simulink subsystem "rss_MotoTempSensFaltDia"  (R2023a)
settings: Solver=VariableStepAuto  StartTime=0.0  StopTime=10.0  RelTol=1e-3
undefined symbols (not defined in the file): ENM_TYPE_FALT, Gu16_ctMotoTempFaltConfCnt_C, Gu16_ctMotoTempFaltRcvyCnt_C, Gu16_uADMotoTempFaltHiLim_C, Gu16_uADMotoTempFaltLoLim_C
libraries: lib_debounce x1, lib_fault_definiteness x1
settings Model: Creator=xiaoqiang.yuan  LastModifiedBy=xiaoqiang.yuan

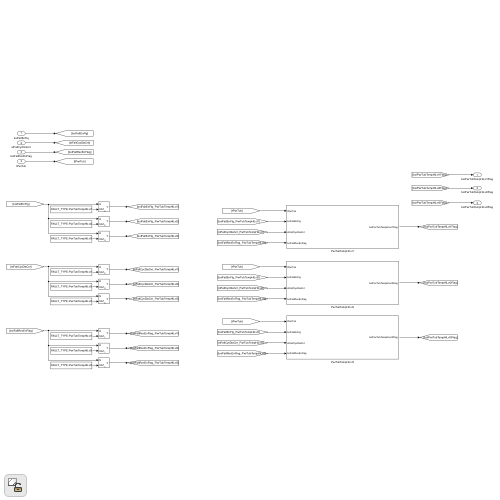
[thumbnail: Simulink's stored preview of the top-level diagram]
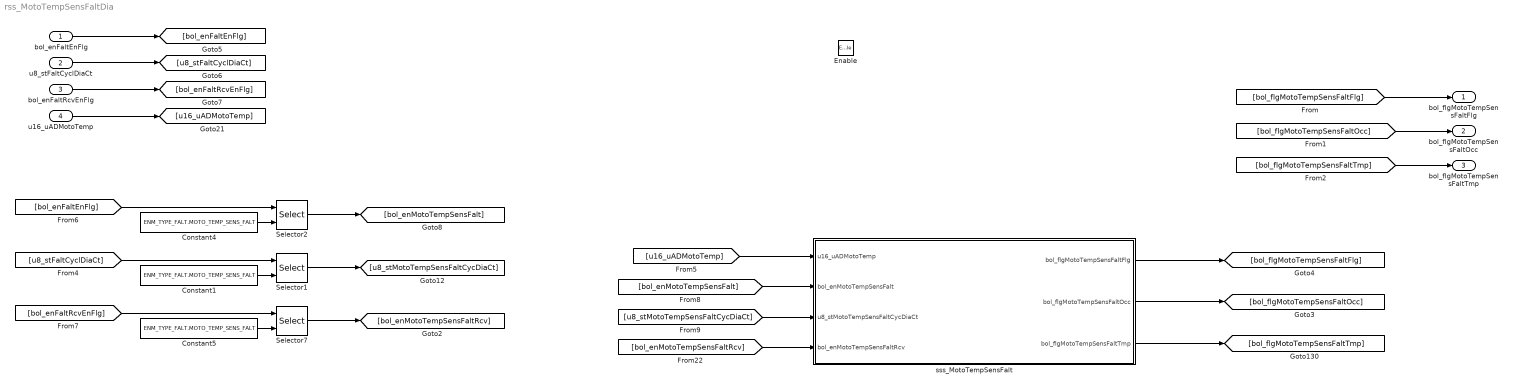
== system rss_MotoTempSensFaltDia ==
  bol_enFaltEnFlg : Inport  OutDataTypeStr=boolean
  u8_stFaltCyclDiaCt : Inport  Port=2  OutDataTypeStr=uint8
  bol_enFaltRcvEnFlg : Inport  Port=3  OutDataTypeStr=boolean
  u16_uADMotoTemp : Inport  Port=4  OutDataTypeStr=uint16
  Enable : EnablePort
  Constant1 : Constant  Value=ENM_TYPE_FALT.MOTO_TEMP_SENS_FALT
  Constant4 : Constant  Value=ENM_TYPE_FALT.MOTO_TEMP_SENS_FALT
  Constant5 : Constant  Value=ENM_TYPE_FALT.MOTO_TEMP_SENS_FALT
  Selector1 : Selector  IndexMode=Zero-based  InputPortWidth=Cdbl_numFaltDiaNum  IndexOptions=Index vector (port)  Indices=[1 3]  OutputSizes=1
  Selector2 : Selector  IndexMode=Zero-based  InputPortWidth=Cdbl_numFaltDiaNum  IndexOptions=Index vector (port)  Indices=[1 3]  OutputSizes=1
  Selector7 : Selector  IndexMode=Zero-based  InputPortWidth=Cdbl_numFaltDiaNum  IndexOptions=Index vector (port)  Indices=[1 3]  OutputSizes=1
  sss_MotoTempSensFalt : Subsystem
  bol_flgMotoTempSensFaltFlg : Outport  OutDataTypeStr=boolean
  bol_flgMotoTempSensFaltOcc : Outport  Port=2  OutDataTypeStr=boolean
  bol_flgMotoTempSensFaltTmp : Outport  Port=3  OutDataTypeStr=boolean
  wires:
  [bol_flgMotoTempSensFaltFlg] -> bol_flgMotoTempSensFaltFlg/1
  u16_uADMotoTemp/1 -> [u16_uADMotoTemp]
  Selector2/1 -> [bol_enMotoTempSensFalt]
  [bol_enFaltEnFlg] -> Selector2/1
  [bol_enMotoTempSensFalt] -> sss_MotoTempSensFalt/2(bol_enMotoTempSensFalt)
  Constant4/1 -> Selector2/2
  [u8_stMotoTempSensFaltCycDiaCt] -> sss_MotoTempSensFalt/3(u8_stMotoTempSensFaltCycDiaCt)
  [u16_uADMotoTemp] -> sss_MotoTempSensFalt/1(u16_uADMotoTemp)
  bol_enFaltEnFlg/1 -> [bol_enFaltEnFlg]
  bol_enFaltRcvEnFlg/1 -> [bol_enFaltRcvEnFlg]
  u8_stFaltCyclDiaCt/1 -> [u8_stFaltCyclDiaCt]
  [bol_enMotoTempSensFaltRcv] -> sss_MotoTempSensFalt/4(bol_enMotoTempSensFaltRcv)
  Selector1/1 -> [u8_stMotoTempSensFaltCycDiaCt]
  Constant1/1 -> Selector1/2
  [u8_stFaltCyclDiaCt] -> Selector1/1
  Selector7/1 -> [bol_enMotoTempSensFaltRcv]
  Constant5/1 -> Selector7/2
  [bol_enFaltRcvEnFlg] -> Selector7/1
  sss_MotoTempSensFalt/1(bol_flgMotoTempSensFaltFlg) -> [bol_flgMotoTempSensFaltFlg]
  sss_MotoTempSensFalt/2(bol_flgMotoTempSensFaltOcc) -> [bol_flgMotoTempSensFaltOcc]
  [bol_flgMotoTempSensFaltOcc] -> bol_flgMotoTempSensFaltOcc/1
  [bol_flgMotoTempSensFaltTmp] -> bol_flgMotoTempSensFaltTmp/1
  sss_MotoTempSensFalt/3(bol_flgMotoTempSensFaltTmp) -> [bol_flgMotoTempSensFaltTmp]

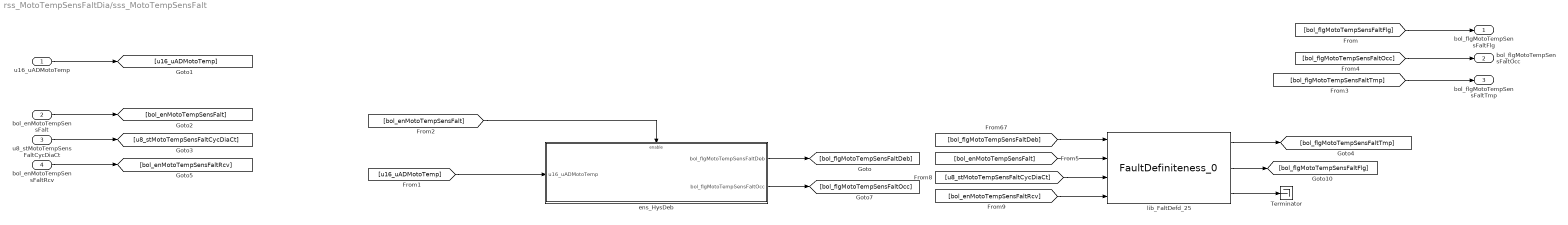
== system rss_MotoTempSensFaltDia/sss_MotoTempSensFalt ==
  u16_uADMotoTemp : Inport
  bol_enMotoTempSensFalt : Inport  Port=2
  u8_stMotoTempSensFaltCycDiaCt : Inport  Port=3
  bol_enMotoTempSensFaltRcv : Inport  Port=4
  Terminator : Terminator
  ens_HysDeb : Subsystem
  lib_FaltDefd_25 : lib_fault_definiteness/FaultDefiniteness_0  lb_FaltWaitRecvCnt=Gu16_ctMotoTempFaltConfCnt_C
  bol_flgMotoTempSensFaltFlg : Outport
  bol_flgMotoTempSensFaltOcc : Outport  Port=2
  bol_flgMotoTempSensFaltTmp : Outport  Port=3  OutDataTypeStr=boolean
  wires:
  [bol_flgMotoTempSensFaltTmp] -> bol_flgMotoTempSensFaltTmp/1
  [bol_flgMotoTempSensFaltOcc] -> bol_flgMotoTempSensFaltOcc/1
  ens_HysDeb/2(bol_flgMotoTempSensFaltOcc) -> [bol_flgMotoTempSensFaltOcc]
  lib_FaltDefd_25/1 -> [bol_flgMotoTempSensFaltTmp]
  lib_FaltDefd_25/2 -> [bol_flgMotoTempSensFaltFlg]
  lib_FaltDefd_25/3 -> Terminator/1
  [bol_enMotoTempSensFalt] -> ens_HysDeb/Enable
  [u16_uADMotoTemp] -> ens_HysDeb/1(u16_uADMotoTemp)
  ens_HysDeb/1(bol_flgMotoTempSensFaltDeb) -> [bol_flgMotoTempSensFaltDeb]
  bol_enMotoTempSensFaltRcv/1 -> [bol_enMotoTempSensFaltRcv]
  u8_stMotoTempSensFaltCycDiaCt/1 -> [u8_stMotoTempSensFaltCycDiaCt]
  bol_enMotoTempSensFalt/1 -> [bol_enMotoTempSensFalt]
  [bol_flgMotoTempSensFaltFlg] -> bol_flgMotoTempSensFaltFlg/1
  u16_uADMotoTemp/1 -> [u16_uADMotoTemp]
  [bol_enMotoTempSensFaltRcv] -> lib_FaltDefd_25/4
  [u8_stMotoTempSensFaltCycDiaCt] -> lib_FaltDefd_25/3
  [bol_enMotoTempSensFalt] -> lib_FaltDefd_25/2
  [bol_flgMotoTempSensFaltDeb] -> lib_FaltDefd_25/1

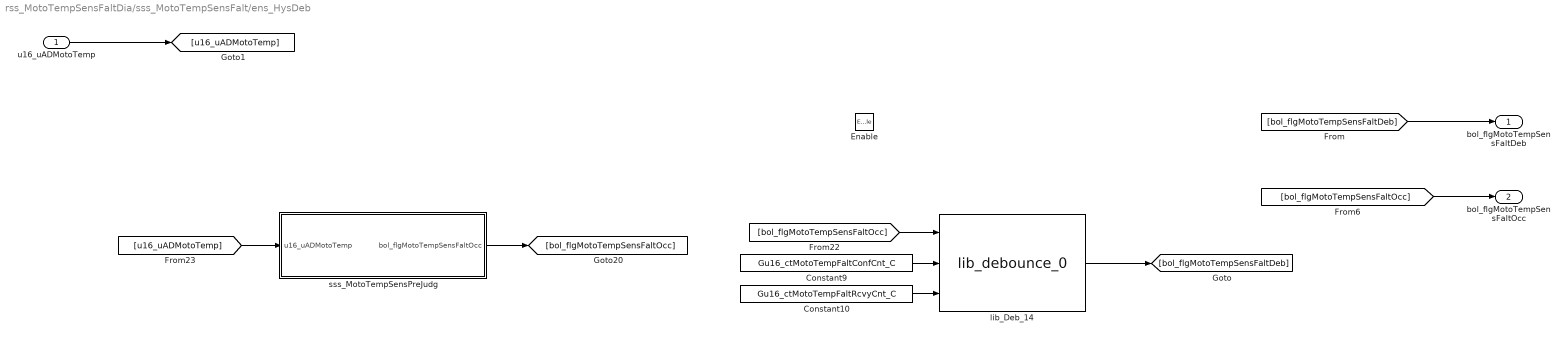
== system rss_MotoTempSensFaltDia/sss_MotoTempSensFalt/ens_HysDeb ==
  u16_uADMotoTemp : Inport
  Enable : EnablePort
  Constant10 : Constant  Value=Gu16_ctMotoTempFaltRcvyCnt_C
  Constant9 : Constant  Value=Gu16_ctMotoTempFaltConfCnt_C
  lib_Deb_14 : lib_debounce/lib_debounce_0
  sss_MotoTempSensPreJudg : Subsystem
  bol_flgMotoTempSensFaltDeb : Outport
  bol_flgMotoTempSensFaltOcc : Outport  Port=2
  wires:
  lib_Deb_14/1 -> [bol_flgMotoTempSensFaltDeb]
  [bol_flgMotoTempSensFaltOcc] -> lib_Deb_14/1
  Constant9/1 -> lib_Deb_14/2
  sss_MotoTempSensPreJudg/1(bol_flgMotoTempSensFaltOcc) -> [bol_flgMotoTempSensFaltOcc]
  Constant10/1 -> lib_Deb_14/3
  [u16_uADMotoTemp] -> sss_MotoTempSensPreJudg/1(u16_uADMotoTemp)
  [bol_flgMotoTempSensFaltOcc] -> bol_flgMotoTempSensFaltOcc/1
  u16_uADMotoTemp/1 -> [u16_uADMotoTemp]
  [bol_flgMotoTempSensFaltDeb] -> bol_flgMotoTempSensFaltDeb/1

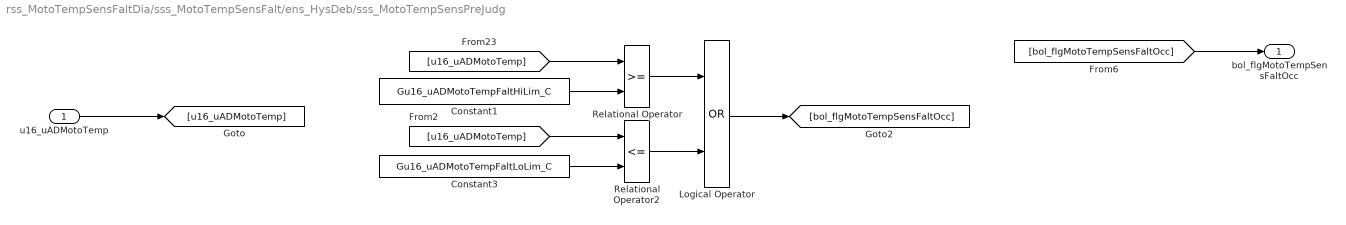
== system rss_MotoTempSensFaltDia/sss_MotoTempSensFalt/ens_HysDeb/sss_MotoTempSensPreJudg ==
  u16_uADMotoTemp : Inport
  Constant1 : Constant  Value=Gu16_uADMotoTempFaltHiLim_C
  Constant3 : Constant  Value=Gu16_uADMotoTempFaltLoLim_C
  Logical Operator : Logic  Operator=OR  AllPortsSameDT=off  OutDataTypeStr=boolean
  Relational Operator : RelationalOperator  OutDataTypeStr=boolean  RndMeth=Simplest  InputSameDT=off
  Relational Operator2 : RelationalOperator  Operator=<=  OutDataTypeStr=boolean  RndMeth=Simplest  InputSameDT=off
  bol_flgMotoTempSensFaltOcc : Outport
  wires:
  u16_uADMotoTemp/1 -> [u16_uADMotoTemp]
  [bol_flgMotoTempSensFaltOcc] -> bol_flgMotoTempSensFaltOcc/1
  Logical Operator/1 -> [bol_flgMotoTempSensFaltOcc]
  Relational Operator2/1 -> Logical Operator/2
  Relational Operator/1 -> Logical Operator/1
  [u16_uADMotoTemp] -> Relational Operator2/1
  Constant3/1 -> Relational Operator2/2
  Constant1/1 -> Relational Operator/2
  [u16_uADMotoTemp] -> Relational Operator/1
